simulink model "Final_Tata_Nexon_EV_Model"  (R2024b)
settings: Solver=VariableStepAuto  StartTime=0.0  StopTime=100
values from neighbouring files (symbols this model uses):
  fault_schedule = [ ... (first row only)    [nexon_params_final.m]
  OCV_col = [300; 318; 330; 341; 355; 375; 403]    [nexon_params_final.m]
  Q_nom = 116    [nexon_params_final.m]
  R_int = 0.12    [nexon_params_final.m]
  SOC_init = 0.8    [nexon_params_final.m]
  SOC_vec = [0, 0.1, 0.25, 0.5, 0.75, 0.9, 1.0]    [nexon_params_final.m]
undefined symbols (not defined in the file or in its folder): canChannel
libraries: canlib x9, canmsglib x8, slpidlib x3, simulink x1
settings Model: SimulationMode=accelerator  NumberOfSteps=10  PacingRate=10  Creator=rtanu  LastModifiedBy=rtanu
settings DebuggingCC: AlgebraicLoopMsg=none

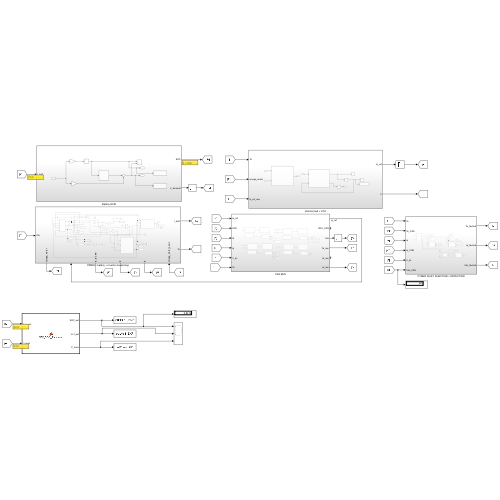
[thumbnail: Simulink's stored preview of the top-level diagram]
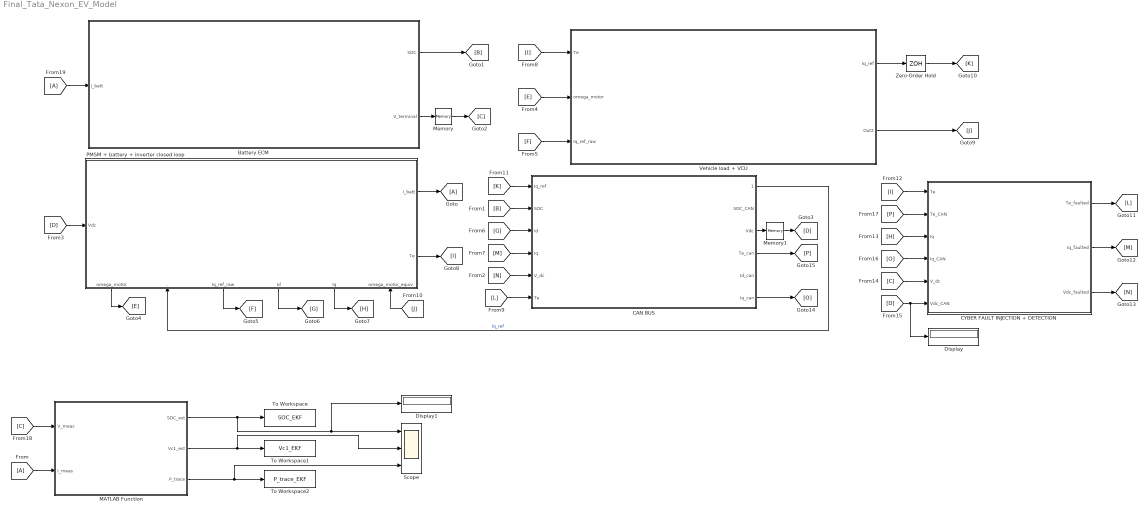
== system Final_Tata_Nexon_EV_Model ==
  Battery ECM : Subsystem
  CAN BUS : Subsystem
  CYBER FAULT INJECTION + DETECTION : Subsystem
  Display : Display
  Display1 : Display
  From : From
  From19 : From
  Goto : Goto
  MATLAB Function : MATLAB Function  TreatAsAtomicUnit=on
  Memory : Memory  InitialCondition=356
  Memory1 : Memory  InitialCondition=356
  PMSM + battery + inverter closed loop : Subsystem
      settings: PortSchema="{\"entries\":[{\"content\":{\"sides\":[{\"content\":{\"connectorIds\":[\"In1\"]},\"type\":\"ConnectorPlacement.EquallySpacedRectSide\",\"uuid\":\"3342cca8-493c-4e30-aa31-ef7ede45f3cb\"},{\"content\":{\"connectorIds\":[\"Out1\",\"Out2\"],\"side\":\"RIGHT\"},\"type\":\"ConnectorPlacement.EquallySpacedRectSide\",\"uuid\":\"986ee4b7-66c5-4e0f-9a1d-6c4d9301284a\"},{\"content\":{\"side\":\"TOP\"},\"type\":\"ConnectorPlacement.EquallySpacedRectSide\",\"uuid\":\"a7ec8491-c75b-4eb8-aca0-0cd4830a82af\"},{\"content\":{\"connectorIds\":[\"Out3\",\"In2\",\"Out4\",\"Out5\",\"Out6\",\"In3\"],\"side\":\"BOTTOM\"},\"type\":\"ConnectorPlacement.EquallySpacedRectSide\",\"uuid\":\"054b5384-e502-435a-a3be-85c80e232110\"}]},\"type\":\"ConnectorPlacement.EquallySpacedConnector\",\"uuid\":\"618faf5e-947e-4e51-9f34-e73e1d551a0f\"}],\"packageUris\":[\"http://schema.mathworks.com/mf0/Connector/R2020b\"],\"version\":\"1.0\"}"
  Scope : Scope  NumInputPorts=3
  To Workspace : ToWorkspace  VariableName=SOC_EKF  SaveFormat=Timeseries  SampleTime=-1
  To Workspace1 : ToWorkspace  VariableName=Vc1_EKF  SaveFormat=Timeseries  SampleTime=-1
  To Workspace2 : ToWorkspace  VariableName=P_trace_EKF  SaveFormat=Timeseries  SampleTime=-1
  Vehicle load + VCU : Subsystem
  Zero-Order Hold : ZeroOrderHold  SampleTime=0.001
  wires:
  PMSM + battery + inverter closed loop/3(omega_motor) -> [E]
  PMSM + battery + inverter closed loop/4(Iq_ref_raw) -> [F]
  Vehicle load + VCU/2(Out2) -> [J]
  Vehicle load + VCU/1(Iq_ref) -> Zero-Order Hold/1
  Zero-Order Hold/1 -> [K]
  CAN BUS/1(" ") -> PMSM + battery + inverter closed loop/2(.)  "Iq_ref"
  Battery ECM/1(SOC) -> [B]
  Battery ECM/2(V_terminal) -> Memory/1
  Memory/1 -> [C]
  CAN BUS/3(Vdc) -> Memory1/1
  PMSM + battery + inverter closed loop/2(Te) -> [I]
  PMSM + battery + inverter closed loop/5(Id) -> [G]
  PMSM + battery + inverter closed loop/6(Iq) -> [H]
  From19/1 -> Battery ECM/1(I_batt)
  PMSM + battery + inverter closed loop/1(I_batt) -> Goto/1
  [B] -> CAN BUS/2(SOC)
  [N] -> CAN BUS/5(V_dc)
  [D] -> PMSM + battery + inverter closed loop/1(Vdc)
  [E] -> Vehicle load + VCU/2(omega_motor)
  [F] -> Vehicle load + VCU/3(Iq_ref_raw)
  [G] -> CAN BUS/3(Id)
  [M] -> CAN BUS/4(Iq)
  [I] -> Vehicle load + VCU/1(Te)
  [J] -> PMSM + battery + inverter closed loop/3(omega_motor_equiv)
  [K] -> CAN BUS/1(Iq_ref)
  Memory1/1 -> [D]
  CYBER FAULT INJECTION + DETECTION/1(Te_faulted) -> [L]
  [L] -> CAN BUS/6(Te)
  [I] -> CYBER FAULT INJECTION + DETECTION/1(Te)
  [H] -> CYBER FAULT INJECTION + DETECTION/3(Iq)
  CYBER FAULT INJECTION + DETECTION/2(Iq_faulted) -> [M]
  [C] -> CYBER FAULT INJECTION + DETECTION/5(V_dc)
  CYBER FAULT INJECTION + DETECTION/3(Vdc_faulted) -> [N]
  [D] -> Display/1, CYBER FAULT INJECTION + DETECTION/6(Vdc_CAN)
  CAN BUS/6(Iq_can) -> [O]
  [O] -> CYBER FAULT INJECTION + DETECTION/4(Iq_CAN)
  CAN BUS/4(Te_can) -> [P]
  [P] -> CYBER FAULT INJECTION + DETECTION/2(Te_CAN)
  From/1 -> MATLAB Function/2(I_meas)
  [C] -> MATLAB Function/1(V_meas)
  MATLAB Function/1(SOC_est) -> Display1/1, Scope/1, To Workspace/1
  MATLAB Function/2(Vc1_est) -> Scope/2, To Workspace1/1
  MATLAB Function/3(P_trace) -> Scope/3, To Workspace2/1

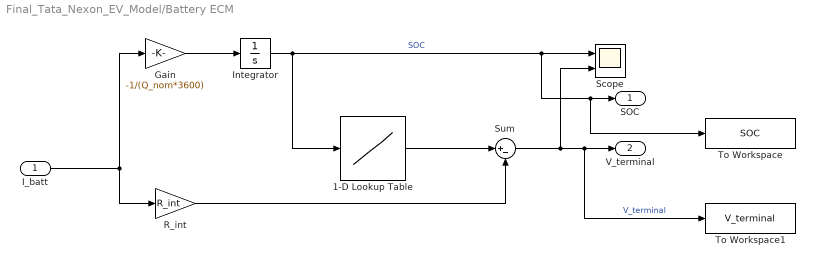
== system Final_Tata_Nexon_EV_Model/Battery ECM ==
  I_batt : Inport
  1-D Lookup Table : Lookup_n-D  NumberOfTableDimensions=1  BreakpointsForDimension1=SOC_vec  Table=OCV_col  InternalRulePriority=Speed  RndMeth=Simplest
  Gain : Gain  Gain=-1/(Q_nom*3600)
  Integrator : Integrator  InitialCondition=SOC_init
  R_int : Gain  Gain=R_int
  Scope : Scope  NumInputPorts=2
  Sum : Sum  Inputs=|+-
  To Workspace : ToWorkspace  VariableName=SOC  SaveFormat=Timeseries  SampleTime=-1
  To Workspace1 : ToWorkspace  VariableName=V_terminal  SaveFormat=Timeseries  SampleTime=-1
  SOC : Outport
  V_terminal : Outport  Port=2
  wires:
  I_batt/1 -> Gain/1, R_int/1
  Integrator/1 -> 1-D Lookup Table/1, To Workspace/1, SOC/1, Scope/1  "SOC"
  Sum/1 -> Scope/2, To Workspace1/1, V_terminal/1  "V_terminal"
  Gain/1 -> Integrator/1
  R_int/1 -> Sum/2
  1-D Lookup Table/1 -> Sum/1

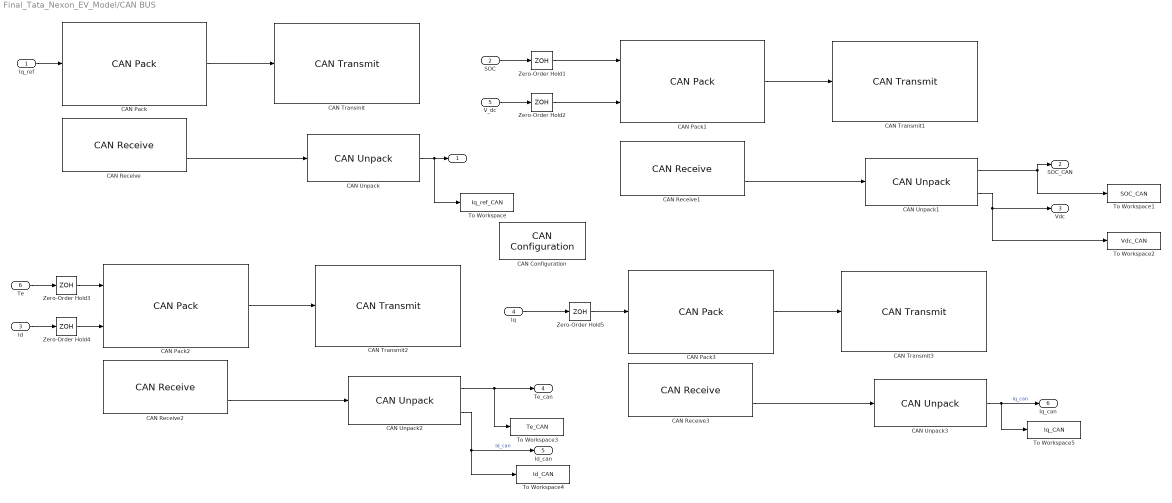
== system Final_Tata_Nexon_EV_Model/CAN BUS ==
  Iq_ref : Inport
  SOC : Inport  Port=2
  Id : Inport  Port=3
  Iq : Inport  Port=4
  V_dc : Inport  Port=5
  Te : Inport  Port=6
  CAN Configuration : canlib/CAN Configuration  BlockHandle=237.0037  Device=MathWorks Virtual 1 (Channel 1)  DeviceMenu=MathWorks Virtual 1 (Channel 1)  ObjConstructor=canChannel('MathWorks', 'Virtual 1', 1)  BusSpeed=500000  EnableBitParameters=off  AckMode=Normal
  CAN Pack : canmsglib/CAN Pack  MsgList=(none)  MsgName=VCU_Command  MsgIDType=Standard (11-bit identifier)  MsgIdentifier=100  CANIDInput=off  MsgLength=8  Remote=off  ApplyMinMax=off  BusOutput=off  SignalInfo={ 'Iq_ref', '0', '32', 'LE', 'signed', 'Standard', '0', '1', '0', '-Inf', 'Inf' }
      settings: DataFormat=manually specified signals
  CAN Pack1 : canmsglib/CAN Pack  MsgList=(none)  MsgName=BMS_Status  MsgIDType=Standard (11-bit identifier)  MsgIdentifier=200  CANIDInput=off  MsgLength=8  Remote=off  ApplyMinMax=off  BusOutput=off  SignalInfo={ 'SOC', '0', '32', 'LE', 'single', 'Standard', '0', '1', '0', '-Inf', 'Inf'; 'V_dc', '32', '32', 'LE', 'signed', 'Standard', '0', '1', '0', '-Inf', 'Inf' }
      settings: DataFormat=manually specified signals
  CAN Pack2 : canmsglib/CAN Pack  MsgList=(none)  MsgName=MCU_te  MsgIDType=Standard (11-bit identifier)  MsgIdentifier=300  CANIDInput=off  MsgLength=8  Remote=off  ApplyMinMax=off  BusOutput=off  SignalInfo={ 'Te', '0', '32', 'LE', 'single', 'Standard', '0', '1', '0', '-Inf', 'Inf'; 'Id', '32', '32', 'LE', 'single', 'Standard', '0', '1', '0', '-Inf', 'Inf' }
      settings: DataFormat=manually specified signals
  CAN Pack3 : canmsglib/CAN Pack  MsgList=(none)  MsgName=MCU_Iq  MsgIDType=Standard (11-bit identifier)  MsgIdentifier=400  CANIDInput=off  MsgLength=8  Remote=off  ApplyMinMax=off  BusOutput=off  SignalInfo={ 'Iq', '0', '32', 'LE', 'single', 'Standard', '0', '1', '0', '-Inf', 'Inf' }
      settings: DataFormat=manually specified signals
  CAN Receive : canlib/CAN Receive  BlockHandle=252.0059  Device=MathWorks Virtual 1 (Channel 1)  DeviceMenu=MathWorks Virtual 1 (Channel 1)  ObjConstructor=canChannel('MathWorks', 'Virtual 1', 1)  EnableStandardIDsFilter=off  StdIDsCombo=Allow all  StandardIDs=0  EnableExtendedIDsFilter=off  ExtIDsCombo=Allow all  ExtendedIDs=0  SampleTime=0.001  MsgsPerTimestep=all  InternalFilterUpdateStatus=on  BusOutput=off
  CAN Receive1 : canlib/CAN Receive  BlockHandle=255.0049  Device=MathWorks Virtual 1 (Channel 1)  DeviceMenu=MathWorks Virtual 1 (Channel 1)  ObjConstructor=canChannel('MathWorks', 'Virtual 1', 1)  EnableStandardIDsFilter=off  StdIDsCombo=Allow all  StandardIDs=0  EnableExtendedIDsFilter=off  ExtIDsCombo=Allow all  ExtendedIDs=0  SampleTime=0.0011  MsgsPerTimestep=all  InternalFilterUpdateStatus=on  BusOutput=off
  CAN Receive2 : canlib/CAN Receive  BlockHandle=258.0027  Device=MathWorks Virtual 1 (Channel 1)  DeviceMenu=MathWorks Virtual 1 (Channel 1)  ObjConstructor=canChannel('MathWorks', 'Virtual 1', 1)  EnableStandardIDsFilter=off  StdIDsCombo=Allow all  StandardIDs=0  EnableExtendedIDsFilter=off  ExtIDsCombo=Allow all  ExtendedIDs=0  SampleTime=0.0012  MsgsPerTimestep=all  InternalFilterUpdateStatus=on  BusOutput=off
  CAN Receive3 : canlib/CAN Receive  BlockHandle=261.0035  Device=MathWorks Virtual 1 (Channel 1)  DeviceMenu=MathWorks Virtual 1 (Channel 1)  ObjConstructor=canChannel('MathWorks', 'Virtual 1', 1)  EnableStandardIDsFilter=off  StdIDsCombo=Allow all  StandardIDs=0  EnableExtendedIDsFilter=off  ExtIDsCombo=Allow all  ExtendedIDs=0  SampleTime=0.00112  MsgsPerTimestep=all  InternalFilterUpdateStatus=on  BusOutput=off
  CAN Transmit : canlib/CAN Transmit  BlockHandle=264.0028  Device=MathWorks Virtual 1 (Channel 1)  DeviceMenu=MathWorks Virtual 1 (Channel 1)  ObjConstructor=canChannel('MathWorks', 'Virtual 1', 1)  EnableEventTransmit=off  EnablePeriodicTransmit=off  MessagePeriod=1.000
  CAN Transmit1 : canlib/CAN Transmit  BlockHandle=266.0027  Device=MathWorks Virtual 1 (Channel 1)  DeviceMenu=MathWorks Virtual 1 (Channel 1)  ObjConstructor=canChannel('MathWorks', 'Virtual 1', 1)  EnableEventTransmit=off  EnablePeriodicTransmit=off  MessagePeriod=1.000
  CAN Transmit2 : canlib/CAN Transmit  BlockHandle=268.0029  Device=MathWorks Virtual 1 (Channel 1)  DeviceMenu=MathWorks Virtual 1 (Channel 1)  ObjConstructor=canChannel('MathWorks', 'Virtual 1', 1)  EnableEventTransmit=off  EnablePeriodicTransmit=off  MessagePeriod=1.000
  CAN Transmit3 : canlib/CAN Transmit  BlockHandle=270.0031  Device=MathWorks Virtual 1 (Channel 1)  DeviceMenu=MathWorks Virtual 1 (Channel 1)  ObjConstructor=canChannel('MathWorks', 'Virtual 1', 1)  EnableEventTransmit=off  EnablePeriodicTransmit=off  MessagePeriod=1.000
  CAN Unpack : canmsglib/CAN Unpack  MsgList=(none)  MsgName=VCU_Command  MsgIDType=Standard (11-bit identifier)  MsgIdentifier=100  MsgLength=8  SignalInfo={ 'Iq_ref', '0', '32', 'LE', 'signed', 'Standard', '0', '1', '0', '-Inf', 'Inf' }  IDPort=off  TimestampPort=off  ErrorPort=off  RemotePort=off  LengthPort=off  StatusPort=off  ApplyMinMax=off
  CAN Unpack1 : canmsglib/CAN Unpack  MsgList=(none)  MsgName=BMS_Status  MsgIDType=Standard (11-bit identifier)  MsgIdentifier=200  MsgLength=8  SignalInfo={ 'SOC', '0', '32', 'LE', 'single', 'Standard', '0', '1', '0', '-Inf', 'Inf'; 'V_dc', '32', '32', 'LE', 'signed', 'Standard', '0', '1', '0', '-Inf', 'Inf' }  IDPort=off  TimestampPort=off  ErrorPort=off  RemotePort=off  LengthPort=off  StatusPort=off  ApplyMinMax=off
  CAN Unpack2 : canmsglib/CAN Unpack  MsgList=(none)  MsgName=MCU_te  MsgIDType=Standard (11-bit identifier)  MsgIdentifier=300  MsgLength=8  SignalInfo={ 'Te', '0', '32', 'LE', 'single', 'Standard', '0', '1', '0', '-Inf', 'Inf'; 'Id', '32', '32', 'LE', 'single', 'Standard', '0', '1', '0', '-Inf', 'Inf' }  IDPort=off  TimestampPort=off  ErrorPort=off  RemotePort=off  LengthPort=off  StatusPort=off  ApplyMinMax=off
  CAN Unpack3 : canmsglib/CAN Unpack  MsgList=(none)  MsgName=MCU_Iq  MsgIDType=Standard (11-bit identifier)  MsgIdentifier=400  MsgLength=8  SignalInfo={ 'Iq', '0', '32', 'LE', 'single', 'Standard', '0', '1', '0', '-Inf', 'Inf' }  IDPort=off  TimestampPort=off  ErrorPort=off  RemotePort=off  LengthPort=off  StatusPort=off  ApplyMinMax=off
  To Workspace : ToWorkspace  VariableName=Iq_ref_CAN  SaveFormat=Timeseries  SampleTime=-1
  To Workspace1 : ToWorkspace  VariableName=SOC_CAN  SaveFormat=Timeseries  SampleTime=-1
  To Workspace2 : ToWorkspace  VariableName=Vdc_CAN  SaveFormat=Timeseries  SampleTime=-1
  To Workspace3 : ToWorkspace  VariableName=Te_CAN  SaveFormat=Timeseries  SampleTime=-1
  To Workspace4 : ToWorkspace  VariableName=Id_CAN  SaveFormat=Timeseries  SampleTime=-1
  To Workspace5 : ToWorkspace  VariableName=Iq_CAN  SaveFormat=Timeseries  SampleTime=-1
  Zero-Order Hold1 : ZeroOrderHold  SampleTime=0.0011
  Zero-Order Hold2 : ZeroOrderHold  SampleTime=0.0011
  Zero-Order Hold3 : ZeroOrderHold  SampleTime=0.0012
  Zero-Order Hold4 : ZeroOrderHold  SampleTime=0.0012
  Zero-Order Hold5 : ZeroOrderHold  SampleTime=0.00112
  " " : Outport
  SOC_CAN : Outport  Port=2
  Vdc : Outport  Port=3
  Te_can : Outport  Port=4
  Id_can : Outport  Port=5
  Iq_can : Outport  Port=6
  wires:
  Id/1 -> Zero-Order Hold4/1
  CAN Unpack1/2 -> To Workspace2/1, Vdc/1
  Zero-Order Hold3/1 -> CAN Pack2/1
  Iq/1 -> Zero-Order Hold5/1
  CAN Receive1/2 -> CAN Unpack1/1
  CAN Receive2/2 -> CAN Unpack2/1
  Zero-Order Hold1/1 -> CAN Pack1/1
  CAN Unpack3/1 -> To Workspace5/1, Iq_can/1  "Iq_can"
  CAN Unpack2/1 -> Te_can/1, To Workspace3/1
  Zero-Order Hold2/1 -> CAN Pack1/2
  SOC/1 -> Zero-Order Hold1/1
  CAN Pack3/1 -> CAN Transmit3/1
  CAN Unpack1/1 -> SOC_CAN/1, To Workspace1/1
  CAN Pack1/1 -> CAN Transmit1/1
  Zero-Order Hold4/1 -> CAN Pack2/2
  Te/1 -> Zero-Order Hold3/1
  CAN Pack2/1 -> CAN Transmit2/1
  CAN Receive3/2 -> CAN Unpack3/1
  CAN Pack/1 -> CAN Transmit/1
  Zero-Order Hold5/1 -> CAN Pack3/1
  CAN Unpack/1 -> To Workspace/1, " "/1
  CAN Unpack2/2 -> Id_can/1, To Workspace4/1  "Id_can"
  Iq_ref/1 -> CAN Pack/1
  CAN Receive/2 -> CAN Unpack/1
  V_dc/1 -> Zero-Order Hold2/1

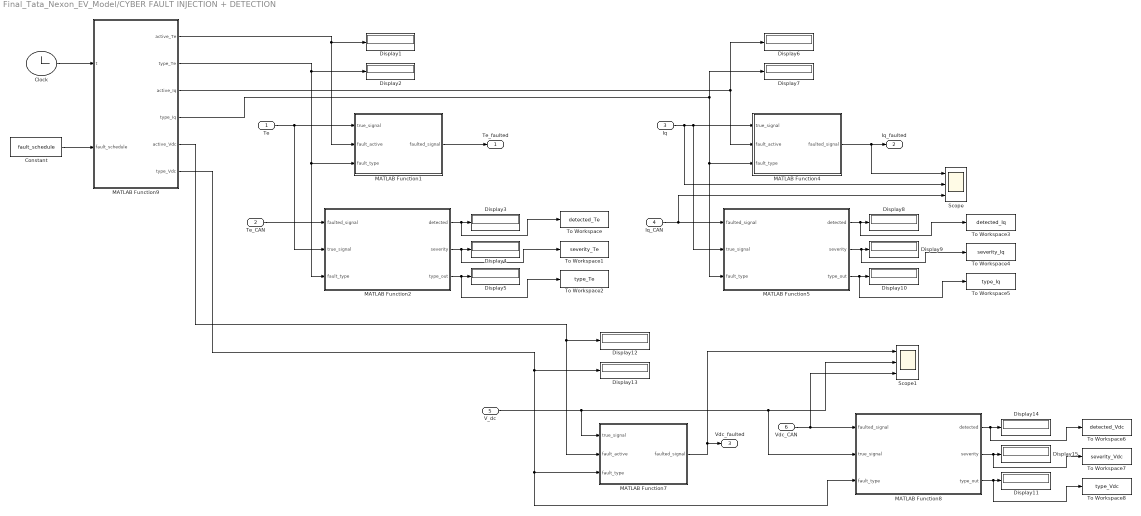
== system Final_Tata_Nexon_EV_Model/CYBER FAULT INJECTION + DETECTION ==
  Te : Inport
  Te_CAN : Inport  Port=2
  Iq : Inport  Port=3
  Iq_CAN : Inport  Port=4
  V_dc : Inport  Port=5
  Vdc_CAN : Inport  Port=6
  Clock : Clock
  Constant : Constant  Value=fault_schedule
  Display{1..15} (15 alike) : Display
  MATLAB Function1 : MATLAB Function  TreatAsAtomicUnit=on
  MATLAB Function2 : MATLAB Function  TreatAsAtomicUnit=on
  MATLAB Function4 : MATLAB Function  TreatAsAtomicUnit=on
  MATLAB Function5 : MATLAB Function  TreatAsAtomicUnit=on
  MATLAB Function7 : MATLAB Function  TreatAsAtomicUnit=on
  MATLAB Function8 : MATLAB Function  TreatAsAtomicUnit=on
  MATLAB Function9 : MATLAB Function  TreatAsAtomicUnit=on
  Scope : Scope  NumInputPorts=3
  Scope1 : Scope  NumInputPorts=3
  To Workspace : ToWorkspace  VariableName=detected_Te  SaveFormat=Timeseries  SampleTime=-1
  To Workspace1 : ToWorkspace  VariableName=severity_Te  SaveFormat=Timeseries  SampleTime=-1
  To Workspace2 : ToWorkspace  VariableName=type_Te  SaveFormat=Timeseries  SampleTime=-1
  To Workspace3 : ToWorkspace  VariableName=detected_Iq  SaveFormat=Timeseries  SampleTime=-1
  To Workspace4 : ToWorkspace  VariableName=severity_Iq  SaveFormat=Timeseries  SampleTime=-1
  To Workspace5 : ToWorkspace  VariableName=type_Iq  SaveFormat=Timeseries  SampleTime=-1
  To Workspace6 : ToWorkspace  VariableName=detected_Vdc  SaveFormat=Timeseries  SampleTime=-1
  To Workspace7 : ToWorkspace  VariableName=severity_Vdc  SaveFormat=Timeseries  SampleTime=-1
  To Workspace8 : ToWorkspace  VariableName=type_Vdc  SaveFormat=Timeseries  SampleTime=-1
  Te_faulted : Outport
  Iq_faulted : Outport  Port=2
  Vdc_faulted : Outport  Port=3
  wires:
  MATLAB Function2/3(type_out) -> To Workspace2/1, Display5/1
  Te/1 -> MATLAB Function2/2(true_signal), MATLAB Function1/1(true_signal)
  MATLAB Function9/1(active_Te) -> MATLAB Function1/2(fault_active), Display1/1
  MATLAB Function2/1(detected) -> To Workspace/1, Display3/1
  MATLAB Function9/2(type_Te) -> MATLAB Function2/3(fault_type), MATLAB Function1/3(fault_type), Display2/1
  MATLAB Function2/2(severity) -> To Workspace1/1, Display4/1
  MATLAB Function1/1(faulted_signal) -> Te_faulted/1
  Te_CAN/1 -> MATLAB Function2/1(faulted_signal)
  MATLAB Function5/1(detected) -> To Workspace3/1, Display8/1
  MATLAB Function9/3(active_Iq) -> Display6/1, MATLAB Function4/2(fault_active)
  MATLAB Function4/1(faulted_signal) -> Scope/1, Iq_faulted/1
  MATLAB Function5/2(severity) -> To Workspace4/1, Display9/1
  MATLAB Function9/4(type_Iq) -> Display7/1, MATLAB Function5/3(fault_type), MATLAB Function4/3(fault_type)
  Iq_CAN/1 -> Scope/3, MATLAB Function5/1(faulted_signal)
  MATLAB Function5/3(type_out) -> To Workspace5/1, Display10/1
  Iq/1 -> Scope/2, MATLAB Function5/2(true_signal), MATLAB Function4/1(true_signal)
  MATLAB Function8/2(severity) -> To Workspace7/1, Display15/1
  V_dc/1 -> MATLAB Function7/1(true_signal), Scope1/2, MATLAB Function8/2(true_signal)
  Vdc_CAN/1 -> Scope1/3, MATLAB Function8/1(faulted_signal)
  MATLAB Function9/6(type_Vdc) -> Display13/1, MATLAB Function7/3(fault_type), MATLAB Function8/3(fault_type)
  MATLAB Function8/3(type_out) -> To Workspace8/1, Display11/1
  MATLAB Function9/5(active_Vdc) -> MATLAB Function7/2(fault_active), Display12/1
  MATLAB Function8/1(detected) -> To Workspace6/1, Display14/1
  MATLAB Function7/1(faulted_signal) -> Scope1/1, Vdc_faulted/1
  Constant/1 -> MATLAB Function9/2(fault_schedule)
  Clock/1 -> MATLAB Function9/1(t)

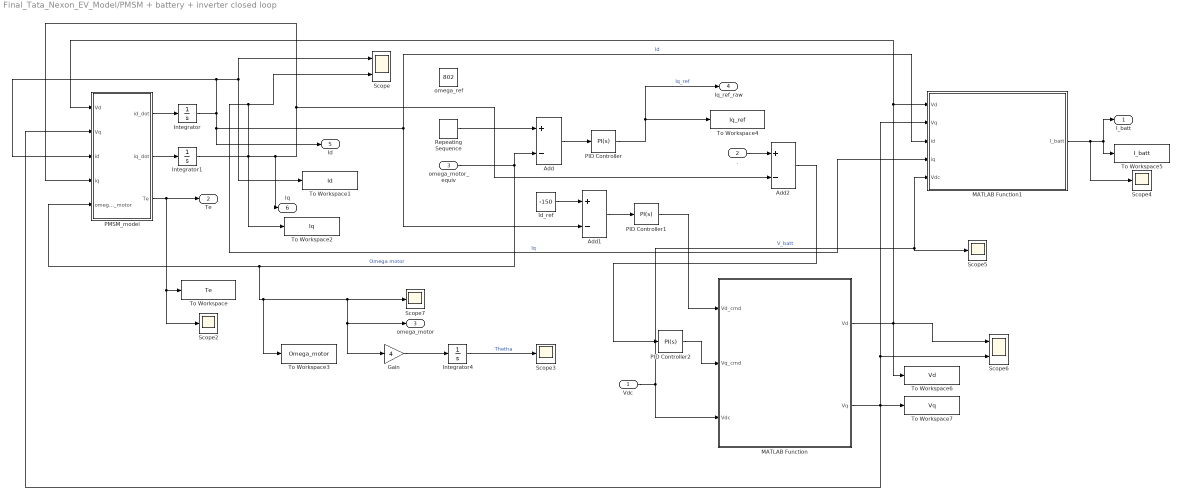
== system Final_Tata_Nexon_EV_Model/PMSM + battery + inverter closed loop ==
  Vdc : Inport
  . : Inport  Port=2
  omega_motor_equiv : Inport  Port=3
  Add : Sum  Inputs=+-
  Add1 : Sum  Inputs=+-
  Add2 : Sum  Inputs=+-
  Gain : Gain  Gain=4
  Id_ref : Constant  Value=-150
  Integrator : Integrator
  Integrator1 : Integrator
  Integrator4 : Integrator  WrapState=on  WrappedStateUpperValue=2*pi  WrappedStateLowerValue=0
  MATLAB Function : MATLAB Function  TreatAsAtomicUnit=on
  MATLAB Function1 : MATLAB Function  TreatAsAtomicUnit=on
  PID Controller : slpidlib/PID Controller  Controller=PI  Form=Parallel  TimeDomain=Continuous-time  UseExternalTs=off  SampleTime=-1  IntegratorMethod=Forward Euler  FilterMethod=Forward Euler  ControllerParametersSource=internal  P=.5  I=2  UseKiTs=off  D=0  UseExternalDerivativeSource=off  N=100  UseFilter=on  TunerSelectOption=Transfer Function Based (PID Tuner App)  InitialConditionSource=internal  InitialConditionForIntegrator=0  InitialConditionForFilter=0  DifferentiatorICPrevScaledInput=0  ExternalReset=none  TrackingMode=off  Kt=1  LimitOutput=on  SatLimitsSource=internal  UpperSaturationLimit=800  LowerSaturationLimit=-800  LinearizeAsGain=on  AntiWindupMode=back-calculation  Kb=1  LimitIntegrator=off  UpperIntegratorSaturationLimit=inf  LowerIntegratorSaturationLimit=-inf  POutMin=[]  POutMax=[]  IOutMin=[]  IOutMax=[]  DOutMin=[]  DOutMax=[]  NOutMin=[]  NOutMax=[]  SumOutMin=[]  SumOutMax=[]  SaturationOutMin=[]  SaturationOutMax=[]  PParamMin=[]  PParamMax=[]  IParamMin=[]  IParamMax=[]  DParamMin=[]  DParamMax=[]  NParamMin=[]  NParamMax=[]  KbParamMin=[]  KbParamMax=[]  KtParamMin=[]  KtParamMax=[]  KbOutMin=[]  KbOutMax=[]  KtOutMin=[]  KtOutMax=[]  IntegratorOutMin=[]  IntegratorOutMax=[]  FilterOutMin=[]  FilterOutMax=[]  SumI1OutMin=[]  SumI1OutMax=[]  SumI2OutMin=[]  SumI2OutMax=[]  SumI3OutMin=[]  SumI3OutMax=[]  SumI4OutMin=[]  SumI4OutMax=[]  SumDOutMin=[]  SumDOutMax=[]  DifferentiatorOutMin=[]  DifferentiatorOutMax=[]  FilterDiffOutCoefMin=[]  FilterDiffOutCoefMax=[]  ReciprocalOutMin=[]  ReciprocalOutMax=[]  SumDenOutMin=[]  SumDenOutMax=[]  SumNumOutMin=[]  SumNumOutMax=[]  DivideOutMin=[]  DivideOutMax=[]  UdiffTsProdOutMin=[]  UdiffTsProdOutMax=[]  NTsProdOutMin=[]  NTsProdOutMax=[]  UintegralTsProdOutMin=[]  UintegralTsProdOutMax=[]  UngainTsProdOutMin=[]  UngainTsProdOutMax=[]  ClampingZeroOutDataTypeStr=Inherit: Inherit via back propagation  ClampingZeroOutMin=[]  ClampingZeroOutMax=[]  FilterDenConstantOutDataTypeStr=Inherit: Inherit via back propagation  FilterDenConstantOutMin=[]  FilterDenConstantOutMax=[]  PCopyOutDataTypeStr=Inherit: Inherit via back propagation  PCopyOutMin=[]  PCopyOutMax=[]  NCopyOutDataTypeStr=Inherit: Inherit via back propagation  NCopyOutMin=[]  NCopyOutMax=[]  IntegratorContinuousStateAttributes=''  IntegratorStateMustResolveToSignalObject=off  IntegratorRTWStateStorageClass=Auto  FilterContinuousStateAttributes=''  FilterStateMustResolveToSignalObject=off  FilterRTWStateStorageClass=Auto  ParallelPVariant=InternalParameters  IdealPVariant=Disabled  IVariant=InternalParameters  DVariant=Disabled  IntegratorVariant=Continuous  SatVariant=Enabled  AWVariant=BackCalculation  PCopyVariant=Disabled  TRVariant=Disabled  FdbkBlocksVariant=Forward  IdealPFdbkVariant=Disabled  SatFdbkVariant=Disabled  DerivativeFilterVariant=Disabled  NVariant=Disabled  NCopyVariant=Disabled_SignalSpec  FilterICVariant=Disabled  IntegratorICVariant=InternalICs  ExternalResetVariant=Disabled  TRSumVariant=Passthrough  SumFdbkVariant=Disabled  SumVariant=Sum_PI  TsampFilterVariant=InternalTs  TsampNgainVariant=Passthrough  TsampIntegralVariant=Disabled_SignalSpec  ExternalSaturationOutDataTypeStr=Inherit: Same as second input  DerivativeSourceVariant=Disabled  PreIntVariant=InternalPreInt
  PID Controller1 : slpidlib/PID Controller  Controller=PI  Form=Parallel  TimeDomain=Continuous-time  UseExternalTs=off  SampleTime=-1  IntegratorMethod=Forward Euler  FilterMethod=Forward Euler  ControllerParametersSource=internal  P=.2  I=20  UseKiTs=off  D=0  UseExternalDerivativeSource=off  N=100  UseFilter=on  TunerSelectOption=Transfer Function Based (PID Tuner App)  InitialConditionSource=internal  InitialConditionForIntegrator=0  InitialConditionForFilter=0  DifferentiatorICPrevScaledInput=0  ExternalReset=none  TrackingMode=off  Kt=1  LimitOutput=on  SatLimitsSource=internal  UpperSaturationLimit=200  LowerSaturationLimit=-200  LinearizeAsGain=on  AntiWindupMode=none  Kb=1  LimitIntegrator=off  UpperIntegratorSaturationLimit=inf  LowerIntegratorSaturationLimit=-inf  POutMin=[]  POutMax=[]  IOutMin=[]  IOutMax=[]  DOutMin=[]  DOutMax=[]  NOutMin=[]  NOutMax=[]  SumOutMin=[]  SumOutMax=[]  SaturationOutMin=[]  SaturationOutMax=[]  PParamMin=[]  PParamMax=[]  IParamMin=[]  IParamMax=[]  DParamMin=[]  DParamMax=[]  NParamMin=[]  NParamMax=[]  KbParamMin=[]  KbParamMax=[]  KtParamMin=[]  KtParamMax=[]  KbOutMin=[]  KbOutMax=[]  KtOutMin=[]  KtOutMax=[]  IntegratorOutMin=[]  IntegratorOutMax=[]  FilterOutMin=[]  FilterOutMax=[]  SumI1OutMin=[]  SumI1OutMax=[]  SumI2OutMin=[]  SumI2OutMax=[]  SumI3OutMin=[]  SumI3OutMax=[]  SumI4OutMin=[]  SumI4OutMax=[]  SumDOutMin=[]  SumDOutMax=[]  DifferentiatorOutMin=[]  DifferentiatorOutMax=[]  FilterDiffOutCoefMin=[]  FilterDiffOutCoefMax=[]  ReciprocalOutMin=[]  ReciprocalOutMax=[]  SumDenOutMin=[]  SumDenOutMax=[]  SumNumOutMin=[]  SumNumOutMax=[]  DivideOutMin=[]  DivideOutMax=[]  UdiffTsProdOutMin=[]  UdiffTsProdOutMax=[]  NTsProdOutMin=[]  NTsProdOutMax=[]  UintegralTsProdOutMin=[]  UintegralTsProdOutMax=[]  UngainTsProdOutMin=[]  UngainTsProdOutMax=[]  ClampingZeroOutDataTypeStr=Inherit: Inherit via back propagation  ClampingZeroOutMin=[]  ClampingZeroOutMax=[]  FilterDenConstantOutDataTypeStr=Inherit: Inherit via back propagation  FilterDenConstantOutMin=[]  FilterDenConstantOutMax=[]  PCopyOutDataTypeStr=Inherit: Inherit via back propagation  PCopyOutMin=[]  PCopyOutMax=[]  NCopyOutDataTypeStr=Inherit: Inherit via back propagation  NCopyOutMin=[]  NCopyOutMax=[]  IntegratorContinuousStateAttributes=''  IntegratorStateMustResolveToSignalObject=off  IntegratorRTWStateStorageClass=Auto  FilterContinuousStateAttributes=''  FilterStateMustResolveToSignalObject=off  FilterRTWStateStorageClass=Auto  ParallelPVariant=InternalParameters  IdealPVariant=Disabled  IVariant=InternalParameters  DVariant=Disabled  IntegratorVariant=Continuous  SatVariant=Enabled  AWVariant=Passthrough  PCopyVariant=Disabled  TRVariant=Disabled  FdbkBlocksVariant=Forward  IdealPFdbkVariant=Disabled  SatFdbkVariant=Disabled  DerivativeFilterVariant=Disabled  NVariant=Disabled  NCopyVariant=Disabled_SignalSpec  FilterICVariant=Disabled  IntegratorICVariant=InternalICs  ExternalResetVariant=Disabled  TRSumVariant=Passthrough  SumFdbkVariant=Disabled  SumVariant=Sum_PI  TsampFilterVariant=InternalTs  TsampNgainVariant=Passthrough  TsampIntegralVariant=Disabled_SignalSpec  ExternalSaturationOutDataTypeStr=Inherit: Same as second input  DerivativeSourceVariant=Disabled  PreIntVariant=InternalPreInt
  PID Controller2 : slpidlib/PID Controller  Controller=PI  Form=Parallel  TimeDomain=Continuous-time  UseExternalTs=off  SampleTime=-1  IntegratorMethod=Forward Euler  FilterMethod=Forward Euler  ControllerParametersSource=internal  P=.2  I=20  UseKiTs=off  D=0  UseExternalDerivativeSource=off  N=100  UseFilter=on  TunerSelectOption=Transfer Function Based (PID Tuner App)  InitialConditionSource=internal  InitialConditionForIntegrator=0  InitialConditionForFilter=0  DifferentiatorICPrevScaledInput=0  ExternalReset=none  TrackingMode=off  Kt=1  LimitOutput=on  SatLimitsSource=internal  UpperSaturationLimit=403  LowerSaturationLimit=-403  LinearizeAsGain=on  AntiWindupMode=none  Kb=1  LimitIntegrator=off  UpperIntegratorSaturationLimit=inf  LowerIntegratorSaturationLimit=-inf  POutMin=[]  POutMax=[]  IOutMin=[]  IOutMax=[]  DOutMin=[]  DOutMax=[]  NOutMin=[]  NOutMax=[]  SumOutMin=[]  SumOutMax=[]  SaturationOutMin=[]  SaturationOutMax=[]  PParamMin=[]  PParamMax=[]  IParamMin=[]  IParamMax=[]  DParamMin=[]  DParamMax=[]  NParamMin=[]  NParamMax=[]  KbParamMin=[]  KbParamMax=[]  KtParamMin=[]  KtParamMax=[]  KbOutMin=[]  KbOutMax=[]  KtOutMin=[]  KtOutMax=[]  IntegratorOutMin=[]  IntegratorOutMax=[]  FilterOutMin=[]  FilterOutMax=[]  SumI1OutMin=[]  SumI1OutMax=[]  SumI2OutMin=[]  SumI2OutMax=[]  SumI3OutMin=[]  SumI3OutMax=[]  SumI4OutMin=[]  SumI4OutMax=[]  SumDOutMin=[]  SumDOutMax=[]  DifferentiatorOutMin=[]  DifferentiatorOutMax=[]  FilterDiffOutCoefMin=[]  FilterDiffOutCoefMax=[]  ReciprocalOutMin=[]  ReciprocalOutMax=[]  SumDenOutMin=[]  SumDenOutMax=[]  SumNumOutMin=[]  SumNumOutMax=[]  DivideOutMin=[]  DivideOutMax=[]  UdiffTsProdOutMin=[]  UdiffTsProdOutMax=[]  NTsProdOutMin=[]  NTsProdOutMax=[]  UintegralTsProdOutMin=[]  UintegralTsProdOutMax=[]  UngainTsProdOutMin=[]  UngainTsProdOutMax=[]  ClampingZeroOutDataTypeStr=Inherit: Inherit via back propagation  ClampingZeroOutMin=[]  ClampingZeroOutMax=[]  FilterDenConstantOutDataTypeStr=Inherit: Inherit via back propagation  FilterDenConstantOutMin=[]  FilterDenConstantOutMax=[]  PCopyOutDataTypeStr=Inherit: Inherit via back propagation  PCopyOutMin=[]  PCopyOutMax=[]  NCopyOutDataTypeStr=Inherit: Inherit via back propagation  NCopyOutMin=[]  NCopyOutMax=[]  IntegratorContinuousStateAttributes=''  IntegratorStateMustResolveToSignalObject=off  IntegratorRTWStateStorageClass=Auto  FilterContinuousStateAttributes=''  FilterStateMustResolveToSignalObject=off  FilterRTWStateStorageClass=Auto  ParallelPVariant=InternalParameters  IdealPVariant=Disabled  IVariant=InternalParameters  DVariant=Disabled  IntegratorVariant=Continuous  SatVariant=Enabled  AWVariant=Passthrough  PCopyVariant=Disabled  TRVariant=Disabled  FdbkBlocksVariant=Forward  IdealPFdbkVariant=Disabled  SatFdbkVariant=Disabled  DerivativeFilterVariant=Disabled  NVariant=Disabled  NCopyVariant=Disabled_SignalSpec  FilterICVariant=Disabled  IntegratorICVariant=InternalICs  ExternalResetVariant=Disabled  TRSumVariant=Passthrough  SumFdbkVariant=Disabled  SumVariant=Sum_PI  TsampFilterVariant=InternalTs  TsampNgainVariant=Passthrough  TsampIntegralVariant=Disabled_SignalSpec  ExternalSaturationOutDataTypeStr=Inherit: Same as second input  DerivativeSourceVariant=Disabled  PreIntVariant=InternalPreInt
  PMSM_model : MATLAB Function  TreatAsAtomicUnit=on
  Repeating Sequence : simulink/Sources/Repeating Sequence  rep_seq_t=[0 8.99 9 12]  rep_seq_y=[802 802 300 300]
  Scope : Scope  NumInputPorts=2
  Scope{2..5,7} (5 alike) : Scope
  Scope6 : Scope  NumInputPorts=2
  To Workspace : ToWorkspace  VariableName=Te  SaveFormat=Timeseries  SampleTime=-1
  To Workspace1 : ToWorkspace  VariableName=Id  SaveFormat=Timeseries  SampleTime=-1
  To Workspace2 : ToWorkspace  VariableName=Iq  SaveFormat=Timeseries  SampleTime=-1
  To Workspace3 : ToWorkspace  VariableName=Omega_motor  SaveFormat=Timeseries  SampleTime=-1
  To Workspace4 : ToWorkspace  VariableName=Iq_ref  SaveFormat=Timeseries  SampleTime=-1
  To Workspace5 : ToWorkspace  VariableName=I_batt  SaveFormat=Timeseries  SampleTime=-1
  To Workspace6 : ToWorkspace  VariableName=Vd  SaveFormat=Timeseries  SampleTime=-1
  To Workspace7 : ToWorkspace  VariableName=Vq  SaveFormat=Timeseries  SampleTime=-1
  omega_ref : Constant  Value=802
  I_batt : Outport
  Te : Outport  Port=2
  omega_motor : Outport  Port=3
  Iq_ref_raw : Outport  Port=4
  Id : Outport  Port=5
  Iq : Outport  Port=6
  wires:
  Integrator/1 -> MATLAB Function1/3(id), Add1/2, Id/1, Scope/1, To Workspace1/1, PMSM_model/3(id)  "Id"
  Id_ref/1 -> Add1/1
  Integrator1/1 -> PMSM_model/4(iq), Add2/2, Iq/1, To Workspace2/1, Scope/2, MATLAB Function1/4(iq)  "Iq"
  MATLAB Function1/1(I_batt) -> I_batt/1, To Workspace5/1, Scope4/1
  PMSM_model/2(iq_dot) -> Integrator1/1
  Add/1 -> PID Controller/1
  Vdc/1 -> MATLAB Function/3(Vdc), MATLAB Function1/5(Vdc), Scope5/1  "V_batt"
  PMSM_model/1(id_dot) -> Integrator/1
  Add1/1 -> PID Controller1/1
  PID Controller1/1 -> MATLAB Function/1(Vd_cmd)
  PID Controller2/1 -> MATLAB Function/2(Vq_cmd)
  PMSM_model/3(Te) -> Te/1, Scope2/1, To Workspace/1
  Add2/1 -> PID Controller2/1
  omega_motor_equiv/1 -> Gain/1, omega_motor/1, Scope7/1, To Workspace3/1, PMSM_model/5(omega_motor), Add/2  "Omega motor"
  Gain/1 -> Integrator4/1
  Integrator4/1 -> Scope3/1  "Thetha"
  PID Controller/1 -> Iq_ref_raw/1, To Workspace4/1  "Iq_ref"
  ./1 -> Add2/1
  Repeating Sequence/1 -> Add/1
  MATLAB Function/1(Vd) -> Scope6/1, PMSM_model/1(Vd), MATLAB Function1/1(Vd), To Workspace6/1
  MATLAB Function/2(Vq) -> PMSM_model/2(Vq), To Workspace7/1, MATLAB Function1/2(Vq), Scope6/2

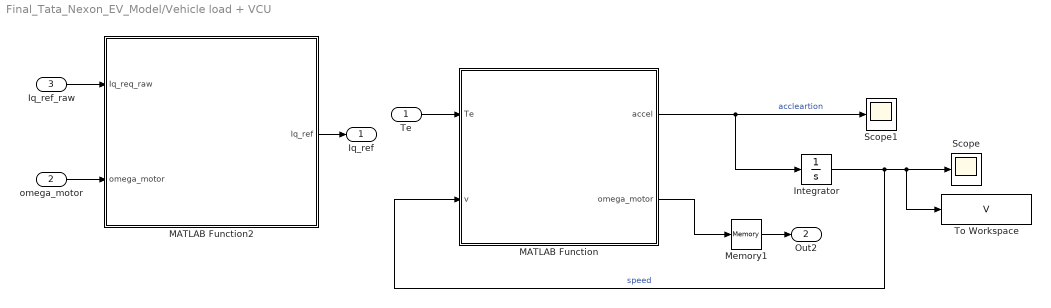
== system Final_Tata_Nexon_EV_Model/Vehicle load + VCU ==
  Te : Inport
  omega_motor : Inport  Port=2
  Iq_ref_raw : Inport  Port=3
  Integrator : Integrator  LimitOutput=on  LowerSaturationLimit=0
  MATLAB Function : MATLAB Function  TreatAsAtomicUnit=on
  MATLAB Function2 : MATLAB Function  TreatAsAtomicUnit=on
  Memory1 : Memory
  Scope : Scope
  Scope1 : Scope
  To Workspace : ToWorkspace  VariableName=V  SaveFormat=Timeseries  SampleTime=-1
  Iq_ref : Outport
  Out2 : Outport  Port=2
  wires:
  MATLAB Function/2(omega_motor) -> Memory1/1
  Integrator/1 -> MATLAB Function/2(v), To Workspace/1, Scope/1  "speed"
  Memory1/1 -> Out2/1
  Iq_ref_raw/1 -> MATLAB Function2/1(Iq_req_raw)
  MATLAB Function/1(accel) -> Scope1/1, Integrator/1  "accleartion"
  omega_motor/1 -> MATLAB Function2/2(omega_motor)
  MATLAB Function2/1(Iq_ref) -> Iq_ref/1
  Te/1 -> MATLAB Function/1(Te)

== matlab function Final_Tata_Nexon_EV_Model/CYBER FAULT INJECTION + DETECTION/MATLAB Function5 ==
  settings: updateMethod=DISCRETE
  data: faulted_signal input; detected output; true_signal input; fault_type input; severity output; type_out output
function [detected, severity, type_out] = fault_detector_Iq(faulted_signal, true_signal, fault_type)
persistent counter
if isempty(counter)
    counter = 0;
end

error_val = abs(faulted_signal - true_signal);

switch fault_type
    case 1,    threshold = 20;   % spoof — offset is 50, so 20 gives clean margin
    case 2,    threshold = 15;   % replay — gap grows over time
    case 3,    threshold = 10;   % dos — signal goes to 0
    case 4,    threshold = 15;   % corruption — noise based
    otherwise, threshold = 20;   % default — conservative
end

if error_val > threshold
    counter = counter + 1;
else
    counter = 0;
end

detected  = counter >= 3;
severity  = error_val;
type_out  = fault_type;
end

== matlab function Final_Tata_Nexon_EV_Model/CYBER FAULT INJECTION + DETECTION/MATLAB Function7 ==
  settings: updateMethod=DISCRETE
  data: true_signal input; faulted_signal output; fault_active input; fault_type input
function faulted_signal = fault_injector_Vdc(true_signal, fault_active, fault_type)
persistent old_value prev_active
if isempty(old_value)
    old_value = true_signal;
end
if isempty(prev_active)
    prev_active = false;
end

% Transition from fault to normal — force clean exit
if prev_active && ~fault_active
    old_value = true_signal;
    faulted_signal = true_signal;
    prev_active = false;
    return;
end

prev_active = fault_active;

if ~fault_active
    old_value = true_signal;
    faulted_signal = true_signal;
    return;
end

switch fault_type
    case 1
        faulted_signal = true_signal + 50;
    case 2
        faulted_signal = old_value;
    case 3
        faulted_signal = 0;
    case 4
        faulted_signal = true_signal + randn()*10;
    otherwise
        faulted_signal = true_signal;
end
end

== matlab function Final_Tata_Nexon_EV_Model/CYBER FAULT INJECTION + DETECTION/MATLAB Function8 ==
  settings: updateMethod=DISCRETE
  data: faulted_signal input; detected output; true_signal input; fault_type input; severity output; type_out output
function [detected, severity, type_out] = fault_detector_Vdc(faulted_signal, true_signal, fault_type)
persistent counter
if isempty(counter)
    counter = 0;
end

error_val = abs(faulted_signal - true_signal);

switch fault_type
    case 1,    threshold = 20;   % spoof — offset is 50, so 20 gives clean margin
    case 2,    threshold = 15;   % replay — gap grows over time
    case 3,    threshold = 10;   % dos — signal goes to 0
    case 4,    threshold = 15;   % corruption — noise based
    otherwise, threshold = 20;   % default — conservative
end

if error_val > threshold
    counter = counter + 1;
else
    counter = 0;
end

detected  = counter >= 3;
severity  = error_val;
type_out  = fault_type;
end

== matlab function Final_Tata_Nexon_EV_Model/CYBER FAULT INJECTION + DETECTION/MATLAB Function9 ==
  data: t input; active_Te output; fault_schedule input; type_Te output; active_Iq output; type_Iq output; active_Vdc output; type_Vdc output
function [active_Te, type_Te, active_Iq, type_Iq, active_Vdc, type_Vdc] = ...
         fault_scheduler(t, fault_schedule)
% Centralized fault scheduler
% Reads fault_schedule matrix, outputs active/type for all 3 signals

active_Te  = false; type_Te  = int32(0);
active_Iq  = false; type_Iq  = int32(0);
active_Vdc = false; type_Vdc = int32(0);

for i = 1:size(fault_schedule, 1)
    sig   = fault_schedule(i,1);
    ftype = fault_schedule(i,2);
    t_s   = fault_schedule(i,3);
    t_e   = fault_schedule(i,4);

    if t >= t_s && t <= t_e
        switch sig
            case 1
                active_Te = true;
                type_Te   = int32(ftype);
            case 2
                active_Iq = true;
                type_Iq   = int32(ftype);
            case 3
                active_Vdc = true;
                type_Vdc   = int32(ftype);
        end
    end
end
end

== matlab function Final_Tata_Nexon_EV_Model/PMSM + battery + inverter closed loop/MATLAB Function ==
  data: Vd_cmd input; Vd output; Vq_cmd input; Vdc input; Vq output
function [Vd, Vq] = voltage_limiter(Vd_cmd, Vq_cmd, Vdc)
% Guard against invalid CAN values from DoS or replay attacks
if Vdc < 50 || Vdc > 450
    Vdc = 350;  % fallback to nominal, simulating BMS protective mode
end

Vmax = Vdc / sqrt(3);
Vmag = sqrt(Vd_cmd^2 + Vq_cmd^2);
if Vmag > Vmax
    scale = Vmax / Vmag;
    Vd = Vd_cmd * scale;
    Vq = Vq_cmd * scale;
else
    Vd = Vd_cmd;
    Vq = Vq_cmd;
end
end

== matlab function Final_Tata_Nexon_EV_Model/MATLAB Function ==
  settings: updateMethod=DISCRETE
  data: V_meas input; SOC_est output; I_meas input; Vc1_est output; P_trace output
function [SOC_est, Vc1_est, P_trace] = EKF_SOC_Estimator(V_meas, I_meas)
%#codegen

persistent x P

% ECM Parameters
R0  = 0.12;
R1  = 0.05;
C1  = 3600;
Q   = 116 * 3600;
dt  = 0.05;

% Noise covariances
Q_n = diag([1e-6, 1e-5]);
R_n = 5.0;   % increased from 0.01 — key change, was too trusting of measurements

% Initialize ONCE with deliberately wrong SOC to show convergence
if isempty(x)
    x = [0.6; 0.0];
    P = diag([0.05, 0.01]);  % larger initial uncertainty
end

% OCV lookup
SOC_bp = [0, 0.05, 0.10, 0.20, 0.30, 0.40, 0.50, ...
          0.60, 0.70, 0.80, 0.90, 0.95, 1.0];
OCV_bp = [280, 303, 315, 325, 331, 336, 341, ...
          346, 352, 362, 378, 390, 403];

%% PREDICT
alpha  = exp(-dt / (R1*C1));
F      = [1, 0; 0, alpha];
B      = [-dt/Q; R1*(1-alpha)];
x_pred = F*x + B*I_meas;
x_pred(1) = max(0.0, min(1.0, x_pred(1)));
P_pred = F*P*F' + Q_n;

%% UPDATE
SOC_c    = max(0.0, min(1.0, x_pred(1)));
OCV_est  = interp1(SOC_bp, OCV_bp, SOC_c, 'linear', 'extrap');

% dOCV/dSOC gradient
d        = 1e-4;
dOCV_dSOC = (interp1(SOC_bp, OCV_bp, min(1,SOC_c+d), 'linear','extrap') - ...
             interp1(SOC_bp, OCV_bp, max(0,SOC_c-d), 'linear','extrap')) / (2*d);

H       = [dOCV_dSOC, -1];
V_pred  = OCV_est - R0*I_meas - x_pred(2);
innov   = V_meas - V_pred;

% Clamp innovation — prevents wild corrections during fault windows
innov   = max(-20, min(20, innov));

S       = H*P_pred*H' + R_n;
K       = P_pred*H' / S;

x       = x_pred + K*innov;
x(1)    = max(0.0, min(1.0, x(1)));

% Joseph form covariance update — numerically stable
I2      = eye(2);
P       = (I2 - K*H)*P_pred*(I2 - K*H)' + K*R_n*K';

%% Outputs
SOC_est = x(1);
Vc1_est = x(2);
P_trace = P(1,1) + P(2,2);

end

== matlab function Final_Tata_Nexon_EV_Model/PMSM + battery + inverter closed loop/PMSM_model ==
  data: Vd input; id_dot output; Vq input; id input; iq input; omega_motor input; iq_dot output; Te output
function [id_dot, iq_dot, Te] = pmsm_model(Vd, Vq, id, iq, omega_motor)
% Electrical-only dq-frame PMSM Model
% Inputs:
%   Vd, Vq      - Stator voltages (V) from voltage_limiter
%   id, iq      - Current states (A) fed back from external integrators
%   omega_motor - Real motor mechanical speed (rad/s) from the vehicle load loop
% Outputs:
%   id_dot, iq_dot - Current derivatives for external integrators
%   Te             - Electromagnetic torque output (Nm)

Ld = 0.0001;     % 100 microhenries (ultra-low for EV high-speed)
Lq = 0.0001;
Rs = 0.015;      % 15 milliohms
lambda = 0.06;   % Lower flux linkage for high-speed overhead

P = 4;

% Electrical d-q differential equations (using electrical rad/s = P * omega_motor)
omega_e = P * omega_motor;

id_dot = (Vd - Rs*id + omega_e * Lq * iq) / Ld;
iq_dot = (Vq - Rs*iq - omega_e * Ld * id - omega_e * lambda) / Lq;

% Electromagnetic torque calculation
Te = 1.5 * P * (lambda * iq + (Ld - Lq) * id * iq);

end

== matlab function Final_Tata_Nexon_EV_Model/PMSM + battery + inverter closed loop/MATLAB Function1 ==
  data: Vd input; I_batt output; Vq input; id input; iq input; Vdc input
function I_batt = battery_current_draw(Vd, Vq, id, iq, Vdc)
P_elec = 1.5 * (Vd*id + Vq*iq);
if Vdc < 50
    I_batt = 0;
    return;
end
I_batt = P_elec / Vdc;
% Physical clamp — Nexon pack max continuous current ~330A
I_batt = max(-330, min(330, I_batt));
end

== matlab function Final_Tata_Nexon_EV_Model/Vehicle load + VCU/MATLAB Function ==
  data: Te input; accel output; v input; omega_motor output
function [accel, omega_motor] = vehicle_load(Te, v)
% Vehicle Longitudinal Dynamics & Rotor Speed Generator
% Inputs:
%   Te - Motor electrical torque (Nm) from pmsm_model
%   v  - Current vehicle speed (m/s) from external v_integrator
% Outputs:
%   accel       - Vehicle acceleration (m/s^2)
%   omega_motor - Real motor speed (rad/s) to drive FOC loop and back-EMF

m_veh   = 1600;
r_wheel = 0.329;
Cd      = 0.29;
A_front = 2.5;
Crr     = 0.012;
rho_air = 1.225;
gear_ratio = 9.5;
g = 9.81;

% Tractive force generated at the tires
F_motor = (Te * gear_ratio) / r_wheel;

% Static/Dynamic rolling resistance ceiling
F_roll_max = Crr * m_veh * g;

% Aerodynamic drag force calculation
F_aero = 0.5 * rho_air * Cd * A_front * v^2 * sign(v);

% Zero-Speed Breakaway Logic
if abs(v) < 1e-4
    if abs(F_motor) <= F_roll_max
        % Motor torque cannot break static friction; vehicle is perfectly stationary
        accel = 0;
    else
        % Motor torque overcomes breakaway threshold
        accel = (F_motor - F_roll_max * sign(F_motor)) / m_veh;
    end
else
    % Vehicle is in motion; rolling resistance opposes the velocity vector
    F_roll = F_roll_max * sign(v);
    F_net = F_motor - F_roll - F_aero;
    accel = F_net / m_veh;
end

% Map the vehicle chassis velocity directly back to motor shaft mechanical speed
omega_motor = (v * gear_ratio) / r_wheel;

end

== matlab function Final_Tata_Nexon_EV_Model/Vehicle load + VCU/MATLAB Function2 ==
  data: Iq_req_raw input; Iq_ref output; omega_motor input
function Iq_ref = vcu_power_limiter(Iq_req_raw, omega_motor)
% Dynamic Constant-Power Torque Limiting
% Inputs:
%   Iq_req_raw  - Raw current requested by Speed PI
%   omega_motor - Mechanical speed of motor (rad/s)
% Outputs:
%   Iq_ref      - Safely bounded Iq target

P_max = 106400; % Nexon EV Max Power: 106.4 kW

% Calculate max physically possible torque at current speed
if abs(omega_motor) < 1
    T_max = 215; % Base torque at standstill
else
    T_max = P_max / abs(omega_motor); % T = Power / speed
    if T_max > 215
        T_max = 215; % Cap at physical motor limit
    end
end

% Convert Torque limit to Iq limit
% Te = 1.5 * P * lambda * Iq  -->  Te = 1.5 * 4 * 0.06 * Iq = 0.36 * Iq
% Iq_max = Te / 0.36
Iq_max = T_max / 0.36;

% Clamp the PI controller's demand to the physical power limit
if Iq_req_raw > Iq_max
    Iq_ref = Iq_max;
elseif Iq_req_raw < -Iq_max
    Iq_ref = -Iq_max;
else
    Iq_ref = Iq_req_raw;
end

end

== matlab function Final_Tata_Nexon_EV_Model/CYBER FAULT INJECTION + DETECTION/MATLAB Function1 ==
  settings: updateMethod=DISCRETE
  data: true_signal input; faulted_signal output; fault_active input; fault_type input
function faulted_signal = fault_injector_Te(true_signal, fault_active, fault_type)
persistent old_value prev_active
if isempty(old_value)
    old_value = true_signal;
end
if isempty(prev_active)
    prev_active = false;
end

% Transition from fault to normal — force clean exit
if prev_active && ~fault_active
    old_value = true_signal;
    faulted_signal = true_signal;
    prev_active = false;
    return;
end

prev_active = fault_active;

if ~fault_active
    old_value = true_signal;
    faulted_signal = true_signal;
    return;
end

switch fault_type
    case 1
        faulted_signal = true_signal + 50;
    case 2
        faulted_signal = old_value;
    case 3
        faulted_signal = 0;
    case 4
        faulted_signal = true_signal + randn()*10;
    otherwise
        faulted_signal = true_signal;
end
end

== matlab function Final_Tata_Nexon_EV_Model/CYBER FAULT INJECTION + DETECTION/MATLAB Function2 ==
  settings: updateMethod=DISCRETE
  data: faulted_signal input; detected output; true_signal input; fault_type input; severity output; type_out output
function [detected, severity, type_out] = fault_detector_Te(faulted_signal, true_signal, fault_type)
persistent counter
if isempty(counter)
    counter = 0;
end

error_val = abs(faulted_signal - true_signal);

switch fault_type
    case 1,    threshold = 20;   % spoof — offset is 50, so 20 gives clean margin
    case 2,    threshold = 15;   % replay — gap grows over time
    case 3,    threshold = 10;   % dos — signal goes to 0
    case 4,    threshold = 15;   % corruption — noise based
    otherwise, threshold = 20;   % default — conservative
end

if error_val > threshold
    counter = counter + 1;
else
    counter = 0;
end

detected  = counter >= 3;
severity  = error_val;
type_out  = fault_type;
end

== matlab function Final_Tata_Nexon_EV_Model/CYBER FAULT INJECTION + DETECTION/MATLAB Function4 ==
  settings: updateMethod=DISCRETE
  data: true_signal input; faulted_signal output; fault_active input; fault_type input
function faulted_signal = fault_injector_Iq(true_signal, fault_active, fault_type)
persistent old_value prev_active
if isempty(old_value)
    old_value = true_signal;
end
if isempty(prev_active)
    prev_active = false;
end

% Transition from fault to normal — force clean exit
if prev_active && ~fault_active
    old_value = true_signal;
    faulted_signal = true_signal;
    prev_active = false;
    return;
end

prev_active = fault_active;

if ~fault_active
    old_value = true_signal;
    faulted_signal = true_signal;
    return;
end

switch fault_type
    case 1
        faulted_signal = true_signal + 50;
    case 2
        faulted_signal = old_value;
    case 3
        faulted_signal = 0;
    case 4
        faulted_signal = true_signal + randn()*10;
    otherwise
        faulted_signal = true_signal;
end
end
